simulink model "VAS_LEVELxTASKx_THT"  (Simulink 3.00)
libraries: paramlib x8, mathlib x6, genlib x4, arclib x2

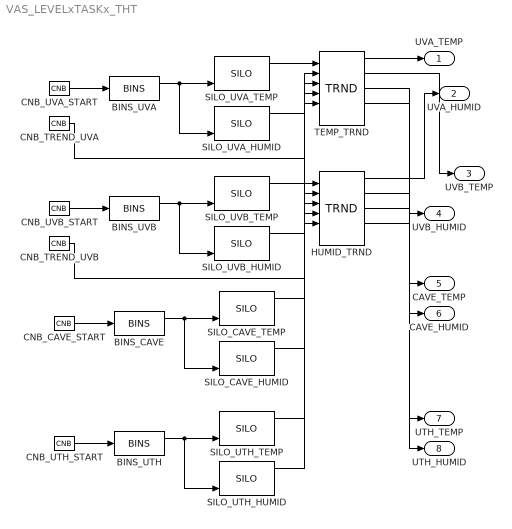
== system VAS_LEVELxTASKx_THT ==
  BINS_CAVE : genlib/BINS  Y0=off  t1=0  t2=1  t3=5  t4=4  t5=5  t6=6  t7=7  t8=8  RPT=on
  BINS_UTH : genlib/BINS  Y0=off  t1=0  t2=1  t3=5  t4=4  t5=5  t6=6  t7=7  t8=8  RPT=on
  BINS_UVA : genlib/BINS  Y0=off  t1=0  t2=1  t3=5  t4=4  t5=5  t6=6  t7=7  t8=8  RPT=on
  BINS_UVB : genlib/BINS  Y0=off  t1=0  t2=1  t3=5  t4=4  t5=5  t6=6  t7=7  t8=8  RPT=on
  CNB_CAVE_START : mathlib/CNB  YCN=on
  CNB_TREND_UVA : mathlib/CNB  YCN=on
  CNB_TREND_UVB : mathlib/CNB  YCN=on
  CNB_UTH_START : mathlib/CNB  YCN=off
  CNB_UVA_START : mathlib/CNB  YCN=on
  CNB_UVB_START : mathlib/CNB  YCN=on
  HUMID_TRND : arclib/TRND  n=3  l=86400  btype=8: Double  ptype1=1: Store  ptype2=1: Store  ptype3=1: Store  ptype4=1: Store  pfac=6  afac=0  arc=0  id=2  Title=HUMIDITY  timesrc=3: RTC
  SILO_CAVE_HUMID : paramlib/SILO  fname=/ramdisk/dht_z3/RH.txt  CSF=off  CLF=off  yerr=0
  SILO_CAVE_TEMP : paramlib/SILO  fname=/ramdisk/dht_z3/TF.txt  CSF=off  CLF=off  yerr=0
  SILO_UTH_HUMID : paramlib/SILO  fname=/ramdisk/dht_z4/RH.txt  CSF=off  CLF=off  yerr=0
  SILO_UTH_TEMP : paramlib/SILO  fname=/ramdisk/dht_z4/TF.txt  CSF=off  CLF=off  yerr=0
  SILO_UVA_HUMID : paramlib/SILO  fname=/ramdisk/dht_z1/RH.txt  CSF=off  CLF=off  yerr=0
  SILO_UVA_TEMP : paramlib/SILO  fname=/ramdisk/dht_z1/TF.txt  CSF=off  CLF=off  yerr=0
  SILO_UVB_HUMID : paramlib/SILO  fname=/ramdisk/dht_z2/RH.txt  CSF=off  CLF=off  yerr=0
  SILO_UVB_TEMP : paramlib/SILO  fname=/ramdisk/dht_z2/TF.txt  CSF=off  CLF=off  yerr=0
  TEMP_TRND : arclib/TRND  n=3  l=86400  btype=8: Double  ptype1=1: Store  ptype2=1: Store  ptype3=1: Store  ptype4=1: Store  pfac=6  afac=0  arc=0  id=1  Title=TEMPERATURE  timesrc=3: RTC
  UVA_TEMP : Outport  Port=1
  UVA_HUMID : Outport  Port=2
  UVB_TEMP : Outport  Port=3
  UVB_HUMID : Outport  Port=4
  CAVE_TEMP : Outport  Port=5
  CAVE_HUMID : Outport  Port=6
  UTH_TEMP : Outport  Port=7
  UTH_HUMID : Outport  Port=8
  wires:
  BINS_CAVE/1 -> SILO_CAVE_HUMID/3, SILO_CAVE_TEMP/3
  BINS_UTH/1 -> SILO_UTH_HUMID/3, SILO_UTH_TEMP/3
  BINS_UVA/1 -> SILO_UVA_HUMID/3, SILO_UVA_TEMP/3
  BINS_UVB/1 -> SILO_UVB_HUMID/3, SILO_UVB_TEMP/3
  CNB_CAVE_START/1 -> BINS_CAVE/1
  CNB_TREND_UVA/1 -> TEMP_TRND/5
  CNB_TREND_UVB/1 -> HUMID_TRND/5
  CNB_UTH_START/1 -> BINS_UTH/1
  CNB_UVA_START/1 -> BINS_UVA/1
  CNB_UVB_START/1 -> BINS_UVB/1
  HUMID_TRND/1 -> UVA_HUMID/1
  HUMID_TRND/2 -> UVB_HUMID/1
  HUMID_TRND/3 -> CAVE_HUMID/1
  HUMID_TRND/4 -> UTH_HUMID/1
  SILO_CAVE_HUMID/1 -> HUMID_TRND/3
  SILO_CAVE_TEMP/1 -> TEMP_TRND/3
  SILO_UTH_HUMID/1 -> HUMID_TRND/4
  SILO_UTH_TEMP/1 -> TEMP_TRND/4
  SILO_UVA_HUMID/1 -> HUMID_TRND/1
  SILO_UVA_TEMP/1 -> TEMP_TRND/1
  SILO_UVB_HUMID/1 -> HUMID_TRND/2
  SILO_UVB_TEMP/1 -> TEMP_TRND/2
  TEMP_TRND/1 -> UVA_TEMP/1
  TEMP_TRND/2 -> UVB_TEMP/1
  TEMP_TRND/3 -> CAVE_TEMP/1
  TEMP_TRND/4 -> UTH_TEMP/1
